simulink model "Bouncing_ball_learn"  (R2017a)
settings: Solver=VariableStepAuto  StartTime=0.0  StopTime=20  MaxStep=1e-3  RelTol=1e-3
libraries: vrlib x2
settings Model: Creator=erich  LastModifiedBy=erich

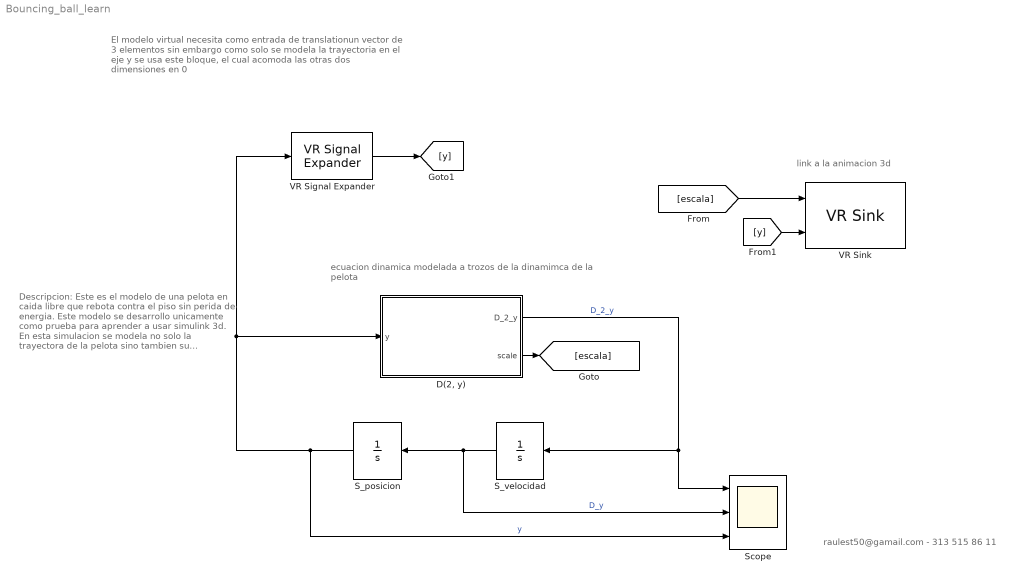
== system Bouncing_ball_learn ==
  note: raulest50@gamail.com - 313 515 86 11
  note: ecuacion dinamica modelada a trozos de
      |  la dinamimca de la pelota
  note: link a la animacion 3d
  note: El modelo virtual necesita como entrada
      | de translationun vector de 3 elementos sin
      | embargo como solo se modela la trayectoria
      | en el eje y se usa este bloque, el cual
      | acomoda las otras dos dimensiones en 0
  note: Descripcion: Este es el modelo
      | de una pelota en caida libre que
      | rebota contra el piso sin
      | perida de energia. Este modelo
      | se desarrollo unicamente como
      | prueba para aprender a usar
      | simulink 3d.
      |
      | En esta simulacion se modela
      | no solo la trayectora de la pelota
      | sino tambien su deformacion.
  "D(2, y)" : MATLAB Function  TreatAsAtomicUnit=on
  S_posicion : Integrator  InitialCondition=20
  S_velocidad : Integrator
  Scope : Scope  NumInputPorts=3
  VR Signal Expander : vrlib/VR Signal Expander  outwidth=3  outidx=[2]
      settings: SourceProductName=Simulink 3D Animation  SourceProductBaseCode=VR
  VR Sink : vrlib/VR Sink  InstantiateOnLoad=on  SampleTime=.005  ViewEnable=on  RemoteChange=off  RemoteView=off  FieldsWritten=Ball.scale.3.1.1.double#Ball.translation.3.1.1.double  WorldFileName=BouncingBall.WRL  AutoView=off  VideoDimensions=[]  AllowVariableSize=off
      settings: SourceProductBaseCode=VR
  wires:
  "D(2, y)"/1(D_2_y) -> Scope/1, S_velocidad/1  "D_2_y"
  S_velocidad/1 -> Scope/2, S_posicion/1  "D_y"
  S_posicion/1 -> Scope/3, VR Signal Expander/1, "D(2, y)"/1(y)  "y"
  "D(2, y)"/2(scale) -> [escala]
  VR Signal Expander/1 -> [y]
  [escala] -> VR Sink/1
  [y] -> VR Sink/2

== matlab function Bouncing_ball_learn/D(2, y) ==
  data: y input; D_2_y output; scale output
function [D_2_y,scale] = fcn(y)
% matlab funciton implementada en simulink 
% para calcular la y'' = f(y). mediante doble integrador
% en simulink se implementa el sistema dinamico y las condiciones
% iniciales.

% D_2_y es la aceleracion en y, el unico eje considerado
% scale corresponde a las longitudes x y z de la esfera cuando se
% se deforma la pelota por choque con el piso.
%  sin deformacion los 3 lados son iguales el radio.
% en el choque se parte de la conservacion del volumen

g = 9.8; % gravedad
K = 50; % coeficiente de elasticidad de la pelota
radio = 1.0;

%en caso de que la posicion de la pelota sea mayor al radio de la
if y>radio % pelota entonces opera la ecuacion de caida libre.
    D_2_y = -g;% la aceleracion es la misma gravedad
    
    % al no tocar el piso, la pelota conserva su forma esferica
    % y por tanto las 3 dimensiones son iguales al radio de la
    % esfera
    scale = [radio radio radio]';
    
else % si la posicion es menor o igual al radio entonces opera esta 
    %ecuacion de elasticidad
    D_2_y = (K*(radio-y))^4 - g;
    %a partir de este momento y es el nuevo radio
    % mientas que las dimensiones horizontales (variable l) 
    % de la es esfera son iguales pero se incrementan 
    % en la medida que y se reduce por conservacion del volumen.
    l = sqrt(radio^3/y);
    scale = [l y l]';
end
